simulink model "LQR"  (R2023b)
settings: Solver=VariableStepAuto  StartTime=0.0  StopTime=20.0  RelTol=1e-3
values from neighbouring files (symbols this model uses):
  A = double(A)    [Rotational_inverted_pendulum.m]
  A_uns = double(A_uns)    [Rotational_inverted_pendulum.m]
  B = double(B)    [Rotational_inverted_pendulum.m]
  B_uns = double(B_uns)    [Rotational_inverted_pendulum.m]
  x1_bar = double(sol.x1)    [Rotational_inverted_pendulum.m]
  x1_bar_uns = x1_bar    [Rotational_inverted_pendulum.m]
  x3_bar = 0    [Rotational_inverted_pendulum.m]
  x3_bar_uns = pi    (= 3.14159265359)    [Rotational_inverted_pendulum.m]
undefined symbols (not defined in the file or in its folder): K_lq, K_lq_uns
libraries: simulink_extras x6, simulink x1
settings Model: Creator=Mark  LastModifiedBy=Mark

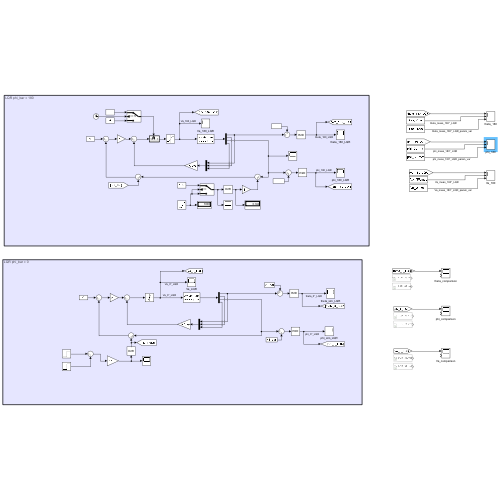
[thumbnail: Simulink's stored preview of the top-level diagram]
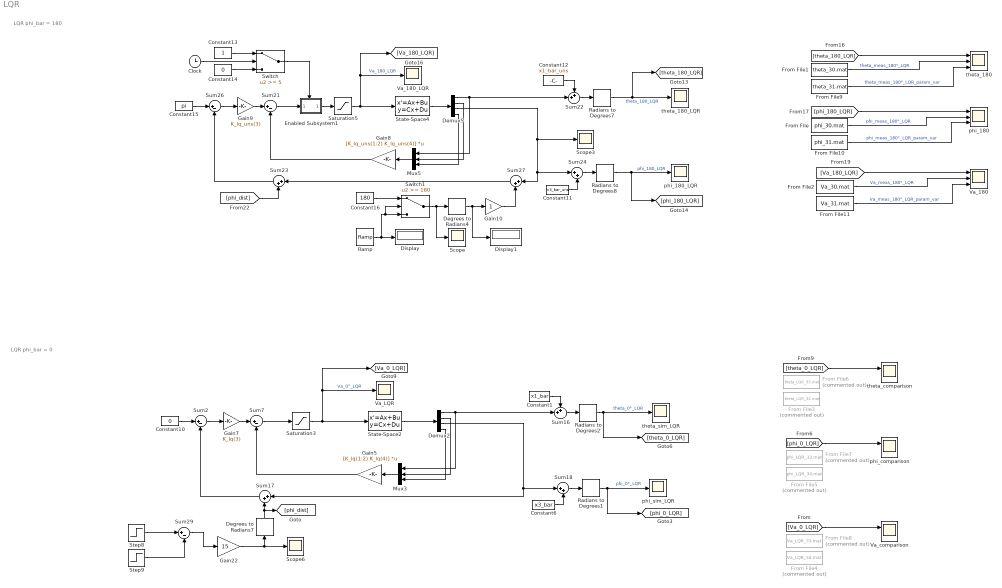
== system LQR ==
  note: LQR phi_bar = 180
  note: LQR phi_bar = 0
  Clock : Clock
  Constant1 : Constant  Value=x1_bar
  Constant10 : Constant  Value=0
  Constant11 : Constant  Value=x3_bar_uns
  Constant12 : Constant  Value=x1_bar_uns
  Constant13 : Constant
  Constant14 : Constant  Value=0
  Constant15 : Constant  Value=pi
  Constant16 : Constant  Value=180
  Constant6 : Constant  Value=x3_bar
  Degrees to Radians4 : simulink_extras/Transformations/Degrees to Radians
  Degrees to Radians7 : simulink_extras/Transformations/Degrees to Radians
  Demux2 : Demux
  Demux5 : Demux
  Display : Display
  Display1 : Display
  Enabled Subsystem1 : Subsystem  TreatAsAtomicUnit=on
  From File : FromFile  FileName=phi_30.mat  SampleTime=0
  From File1 : FromFile  FileName=theta_30.mat  SampleTime=0
  From File10 : FromFile  FileName=phi_31.mat  SampleTime=0
  From File11 : FromFile  FileName=Va_31.mat  SampleTime=0
  From File2 : FromFile  FileName=Va_30.mat  SampleTime=0
  From File3 : FromFile  Commented=on  FileName=theta_LQR_34.mat  SampleTime=0
  From File4 : FromFile  Commented=on  FileName=Va_LQR_34.mat  SampleTime=0
  From File5 : FromFile  Commented=on  FileName=phi_LQR_34.mat  SampleTime=0
  From File6 : FromFile  Commented=on  FileName=theta_LQR_33.mat  SampleTime=0
  From File7 : FromFile  Commented=on  FileName=phi_LQR_33.mat  SampleTime=0
  From File8 : FromFile  Commented=on  FileName=Va_LQR_33.mat  SampleTime=0
  From File9 : FromFile  FileName=theta_31.mat  SampleTime=0
  Gain10 : Gain
  Gain22 : Gain  Gain=15
  Gain5 : Gain  Gain=[K_lq(1:2) K_lq(4)]  Multiplication=Matrix(K*u) (u vector)
  Gain7 : Gain  Gain=K_lq(3)
  Gain8 : Gain  Gain=[K_lq_uns(1:2) K_lq_uns(4)]  Multiplication=Matrix(K*u) (u vector)
  Gain9 : Gain  Gain=K_lq_uns(3)
  Mux3 : Mux  Inputs=3
  Mux5 : Mux  Inputs=3
  Radians to Degrees{1..2,7..8} (4 alike) : simulink_extras/Transformations/Radians to Degrees
  Ramp : simulink/Sources/Ramp  slope=50  start=0  InitialOutput=0
  Saturation3 : Saturate  UpperLimit=10  LowerLimit=-10
  Saturation5 : Saturate  UpperLimit=10  LowerLimit=-10
  Scope : Scope
  Scope3 : Scope
  Scope6 : Scope
  State-Space2 : StateSpace  A=A  B=B  C=eye(4)  D=zeros(4,1)  InitialCondition=[0 0 0 0]
  State-Space4 : StateSpace  A=A_uns  B=B_uns  C=eye(4)  D=zeros(4,1)  InitialCondition=[ 0 0 0 0]
  Step8 : Step  Time=10  SampleTime=0
  Step9 : Step  Time=10.05  SampleTime=0
  Sum16 : Sum  Inputs=++|
  Sum{17..18,23..24,27} (5 alike) : Sum  Inputs=|++
  Sum{2,7,21,26,29} (5 alike) : Sum  Inputs=|+-
  Sum22 : Sum  Inputs=++|
  Switch : Switch  Threshold=5  SaturateOnIntegerOverflow=off  InputSameDT=off
  Switch1 : Switch  Threshold=180  SaturateOnIntegerOverflow=off  InputSameDT=off
  Va_180 : Scope  NumInputPorts=3
  Va_180_LQR : Scope
  Va_LQR : Scope
  Va_comparison : Scope  NumInputPorts=2
  phi_180 : Scope  NumInputPorts=3
  phi_180_LQR : Scope
  phi_comparison : Scope  NumInputPorts=2
  phi_sim_LQR : Scope
  theta_180 : Scope  NumInputPorts=3
  theta_180_LQR : Scope
  theta_comparison : Scope  NumInputPorts=2
  theta_sim_LQR : Scope
  wires:
  Constant15/1 -> Sum26/1
  Mux5/1 -> Gain8/1
  Constant12/1 -> Sum22/1
  Saturation5/1 -> State-Space4/1, Va_180_LQR/1, [Va_180_LQR]  "Va_180_LQR"
  Sum21/1 -> Enabled Subsystem1/1(In1)
  Demux5/3 -> Scope3/1, Sum27/1, Sum24/1
  Sum22/1 -> Radians to Degrees7/1
  Constant11/1 -> Sum24/2
  Ramp/1 -> Switch1/2, Switch1/3, Display/1
  Gain9/1 -> Sum21/1
  Switch1/1 -> Scope/1, Degrees to Radians4/1
  Enabled Subsystem1/1(Out1) -> Saturation5/1
  State-Space4/1 -> Demux5/1
  Radians to Degrees7/1 -> [theta_180_LQR], theta_180_LQR/1  "theta_180_LQR"
  Constant16/1 -> Switch1/1
  Demux5/4 -> Mux5/3
  Sum27/1 -> Sum23/1
  [phi_dist] -> Sum23/2
  Sum24/1 -> Radians to Degrees8/1
  Sum23/1 -> Sum26/2
  Constant13/1 -> Switch/1
  Demux5/1 -> Sum22/2, Mux5/1
  Constant14/1 -> Switch/3
  Degrees to Radians4/1 -> Display1/1, Gain10/1
  Switch/1 -> Enabled Subsystem1/Enable
  Sum26/1 -> Gain9/1
  Gain8/1 -> Sum21/2
  Clock/1 -> Switch/2
  Demux5/2 -> Mux5/2
  Gain10/1 -> Sum27/2
  Radians to Degrees8/1 -> [phi_180_LQR], phi_180_LQR/1  "phi_180_LQR"
  Constant6/1 -> Sum18/2
  Saturation3/1 -> State-Space2/1, [Va_0_LQR], Va_LQR/1  "Va_0°_LQR"
  Constant10/1 -> Sum2/1
  Gain7/1 -> Sum7/1
  Radians to Degrees2/1 -> theta_sim_LQR/1, [theta_0_LQR]  "theta_0°_LQR"
  Radians to Degrees1/1 -> [phi_0_LQR], phi_sim_LQR/1  "phi_0°_LQR"
  Demux2/3 -> Sum17/1, Sum18/1
  Demux2/4 -> Mux3/3
  Sum18/1 -> Radians to Degrees1/1
  Gain5/1 -> Sum7/2
  Demux2/1 -> Sum16/2, Mux3/1
  Demux2/2 -> Mux3/2
  Mux3/1 -> Gain5/1
  Sum16/1 -> Radians to Degrees2/1
  Sum7/1 -> Saturation3/1
  Sum2/1 -> Gain7/1
  State-Space2/1 -> Demux2/1
  Constant1/1 -> Sum16/1
  Sum17/1 -> Sum2/2
  [phi_180_LQR] -> phi_180/1
  From File1/1 -> theta_180/2  "theta_meas_180°_LQR"
  [Va_180_LQR] -> Va_180/1
  [theta_180_LQR] -> theta_180/1
  From File2/1 -> Va_180/2  "Va_meas_180°_LQR"
  From File/1 -> phi_180/2  "phi_meas_180°_LQR"
  [phi_0_LQR] -> phi_comparison/1
  [theta_0_LQR] -> theta_comparison/1
  [Va_0_LQR] -> Va_comparison/1
  Step8/1 -> Sum29/1
  Gain22/1 -> Scope6/1, Degrees to Radians7/1
  Step9/1 -> Sum29/2
  Sum29/1 -> Gain22/1
  Degrees to Radians7/1 -> [phi_dist], Sum17/2
  From File9/1 -> theta_180/3  "theta_meas_180°_LQR_param_var"
  From File10/1 -> phi_180/3  "phi_meas_180°_LQR_param_var"
  From File11/1 -> Va_180/3  "Va_meas_180°_LQR_param_var"

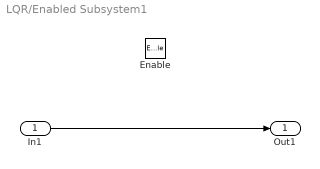
== system LQR/Enabled Subsystem1 ==
  In1 : Inport
  Enable : EnablePort
  Out1 : Outport
  wires:
  In1/1 -> Out1/1
